simulink model "board_virgin_lab4"  (R2015a)
settings: Solver=ode3  StartTime=0.0  StopTime=inf  FixedStep=0.001  RelTol=1e-3
values from neighbouring files (symbols this model uses):
  PID_sim = PID(12)    [callback.m]    (also in postproc_lab04.m = PID(PID_idx(ii)))
  ref_2 = [0 0]    [callback.m]
  ref_3 = [0.09 0.07]    [callback.m]
  T1gain = Pt1(1)    [callback.m]
  T1offset = Pt1(2)    [callback.m]
  T2gain = Pt2(1)    [callback.m]
  T2offset = Pt2(2)    [callback.m]
  Xgain = Px(1)    [callback.m]
  Xoffset = Px(2)    [callback.m]
  Xtare_raw = [870 1250 2036 2836 3410]    [callback.m]
  Xtare_real = [-127.5 -80 0 80 127.5] * 1e-3    [callback.m]
  Ygain = Py(1)    [callback.m]
  Yoffset = Py(2)    [callback.m]
  Ytare_raw = [890 1370 2040 2690 3409]    [callback.m]
  Ytare_real = [-97.5 -50 0 50 110]*1e-3    [callback.m]
libraries: PoliArd x14, simulink x6, simulink_extras x1, dspsigops x1
settings Model: ExtModeTrigDuration=2  Creator=User  LastModifiedBy=user
settings OptimizationCC: OptimizeModelRefInitCode=on  LifeSpan=1
settings DebuggingCC: UnderspecifiedInitializationDetection=Classic  MergeDetectMultiDrivingBlocksExec=none
settings HardwareCC: ProdLargestAtomicInteger=Long  ProdLargestAtomicFloat=Double  ProdEndianess=LittleEndian  ProdHWDeviceType=ARM Compatible->ARM Cortex
settings RTWCC: SystemTargetFile=realtime.tlc  GenerateMakefile=off  TemplateMakefile=realtime.tmf  Description=Run on Target Hardware  RTWVerbose=off
settings ERTTargetCC: CombineOutputUpdateFcns=off  ExtModeTransport=3  ExtModeMexFile=ext_serial_win32_comm_rtt  ExtModeMexArgs=0 1 9600  InlinedParameterPlacement=Hierarchical  ERTSrcFileBannerTemplate=realtime_code_template.cgt  ERTHdrFileBannerTemplate=realtime_code_template.cgt  ERTDataSrcFileTemplate=realtime_code_template.cgt  ERTDataHdrFileTemplate=realtime_code_template.cgt  ERTCustomFileTemplate=realtime_file_process.tlc

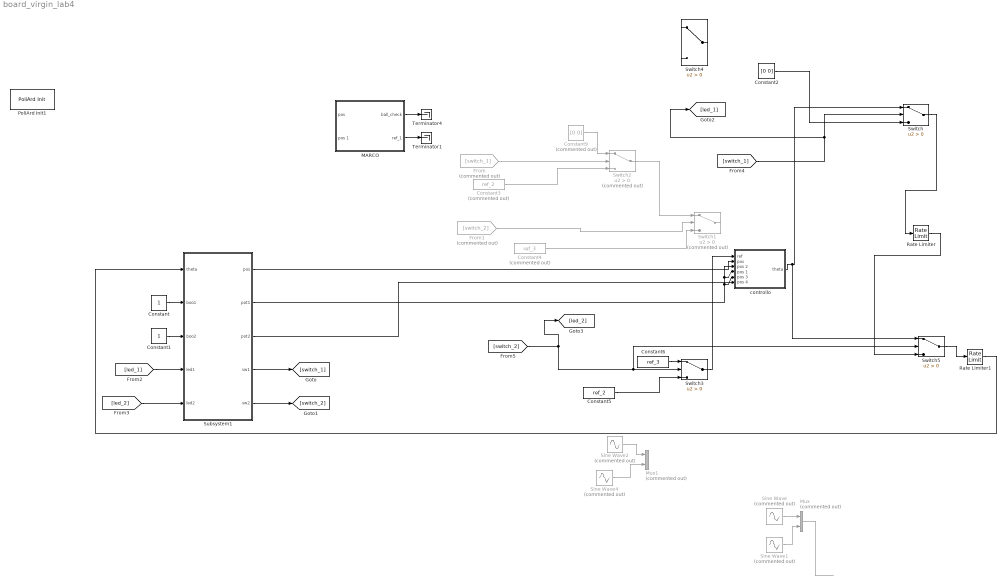
== system board_virgin_lab4 ==
  Constant : Constant  SampleTime=0.01
  Constant1 : Constant  SampleTime=0.01
  Constant2 : Constant  Value=[0 0]
  Constant3 : Constant  Commented=on  Value=ref_2
  Constant4 : Constant  Commented=on  Value=ref_3
  Constant5 : Constant  Value=ref_2
  Constant6 : Constant  Value=ref_3
  Constant9 : Constant  Commented=on  Value=[0 0]
  From : From  Commented=on  GotoTag=switch_1
  From1 : From  Commented=on  GotoTag=switch_2
  MARCO : Subsystem
  Mux : Mux  Commented=on  Inputs=2
  Mux1 : Mux  Commented=on  Inputs=2
  PoliArd Init1 : PoliArd/PoliArd Init
  Rate Limiter : RateLimiter  RisingSlewLimit=20  FallingSlewLimit=-20  SampleTimeMode=inherited
  Rate Limiter1 : RateLimiter  RisingSlewLimit=20  FallingSlewLimit=-20  SampleTimeMode=inherited
  Sine Wave : Sin  Commented=on  SampleTime=0
  Sine Wave1 : Sin  Commented=on  Phase=pi/2  SampleTime=0
  Sine Wave2 : Sin  Commented=on  Amplitude=0.03  Frequency=2*pi*0.1  SampleTime=0
  Sine Wave4 : Sin  Commented=on  Amplitude=0.03  Frequency=2*pi*0.1  Phase=pi/2  SampleTime=0
  Subsystem1 : Subsystem
  Switch{,3..5} (4 alike) : Switch  Criteria=u2 > Threshold
  Switch1 : Switch  Commented=on  Criteria=u2 > Threshold
  Switch2 : Switch  Commented=on  Criteria=u2 > Threshold
  Terminator1 : Terminator
  Terminator4 : Terminator
  "controllo " : Subsystem  SystemSampleTime=0.01
  wires:
  Subsystem1/1("pos ") -> "controllo "/2("pos ")
  Subsystem1/4(sw1) -> [switch_1]
  Subsystem1/5(sw2) -> [switch_2]
  From/1 -> Switch2/2
  From1/1 -> Switch1/2
  Constant4/1 -> Switch1/3
  [led_1] -> Subsystem1/4("led1 ")
  Constant/1 -> Subsystem1/2(boo1)
  Constant1/1 -> Subsystem1/3(boo2)
  [led_2] -> Subsystem1/5(led2)
  Constant3/1 -> Switch2/3
  Switch2/1 -> Switch1/1
  MARCO/2(ref_1) -> Terminator1/1
  Constant9/1 -> Switch2/1
  [switch_1] -> Switch/2, [led_1]
  MARCO/1(ball_check) -> Terminator4/1
  Constant2/1 -> Switch/3
  "controllo "/1(theta) -> Switch5/1, Switch/1
  Switch/1 -> Rate Limiter/1
  [switch_2] -> [led_2], Switch5/2, Switch3/2
  Constant5/1 -> Switch3/3
  Switch3/1 -> "controllo "/1("ref ")
  Rate Limiter/1 -> Switch5/3
  Switch5/1 -> Rate Limiter1/1
  Rate Limiter1/1 -> Subsystem1/1(theta)
  Mux/1 -> ?
  Sine Wave/1 -> Mux/1
  Sine Wave1/1 -> Mux/2
  Subsystem1/2(pot1) -> "controllo "/4(pos 1), "controllo "/3(pos 2), "controllo "/5(pos 3)
  Subsystem1/3(pot2) -> "controllo "/6(pos 4)
  Sine Wave2/1 -> Mux1/1
  Sine Wave4/1 -> Mux1/2
  Constant6/1 -> Switch3/1

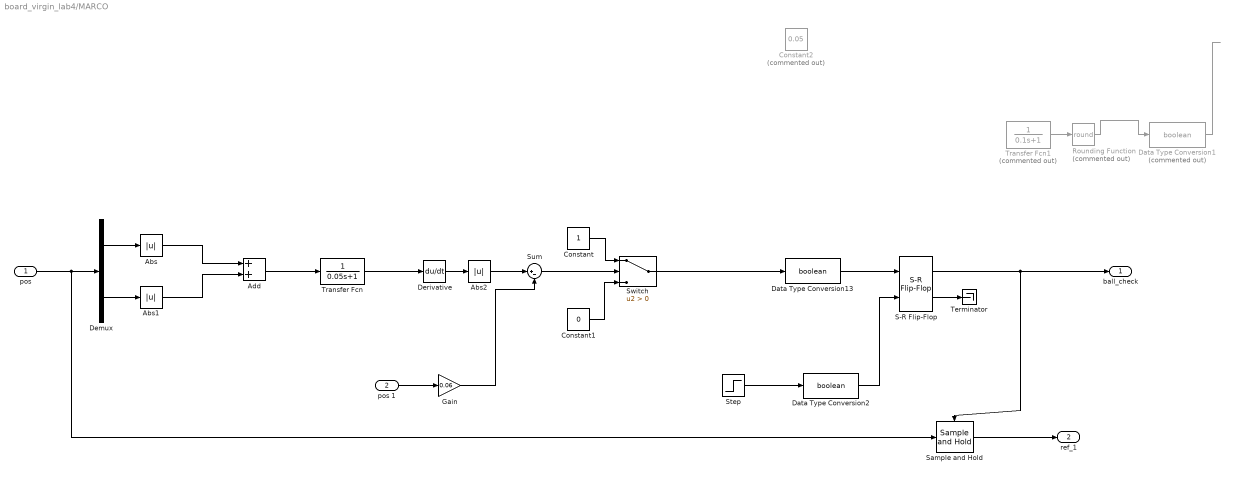
== system board_virgin_lab4/MARCO ==
  "pos " : Inport
  pos 1 : Inport  Port=2
  Abs : Abs
  Abs1 : Abs
  Abs2 : Abs
  Add : Sum
  Constant : Constant
  Constant1 : Constant  Value=0
  Constant2 : Constant  Commented=on  Value=0.05
  Data Type Conversion1 : DataTypeConversion  Commented=on  OutDataTypeStr=boolean
  Data Type Conversion13 : DataTypeConversion  OutDataTypeStr=boolean
  Data Type Conversion2 : DataTypeConversion  OutDataTypeStr=boolean
  Demux : Demux  Outputs=2
  Derivative : Derivative
  Gain : Gain  Gain=0.06
  Rounding Function : Rounding  Commented=on  Operator=round
  S-R Flip-Flop : simulink_extras/Flip Flops/S-R Flip-Flop  initial_condition=0
  Sample and Hold : dspsigops/Sample and Hold  trig=Rising edge  initCond=0  latchinput=off
  Step : Step  Before=1  After=0
  Sum : Sum  Inputs=|+-
  Switch : Switch  Criteria=u2 > Threshold
  Terminator : Terminator
  Transfer Fcn : TransferFcn  Denominator=[0.05 1]
  Transfer Fcn1 : TransferFcn  Commented=on  Denominator=[0.1 1]
  ball_check : Outport
  ref_1 : Outport  Port=2
  wires:
  "pos "/1 -> Sample and Hold/1, Demux/1
  Demux/1 -> Abs/1
  Demux/2 -> Abs1/1
  Abs1/1 -> Add/2
  Abs/1 -> Add/1
  Derivative/1 -> Abs2/1
  Abs2/1 -> Sum/1
  Sum/1 -> Switch/2
  Constant/1 -> Switch/1
  Constant1/1 -> Switch/3
  Sample and Hold/1 -> ref_1/1
  Add/1 -> Transfer Fcn/1
  Transfer Fcn/1 -> Derivative/1
  Gain/1 -> Sum/2
  S-R Flip-Flop/1 -> ball_check/1, Sample and Hold/Trigger
  S-R Flip-Flop/2 -> Terminator/1
  Data Type Conversion13/1 -> S-R Flip-Flop/1
  Switch/1 -> Data Type Conversion13/1
  Transfer Fcn1/1 -> Rounding Function/1
  Rounding Function/1 -> Data Type Conversion1/1
  ? -> Transfer Fcn1/1
  Data Type Conversion1/1 -> ?
  Data Type Conversion2/1 -> S-R Flip-Flop/2
  Step/1 -> Data Type Conversion2/1
  pos 1/1 -> Gain/1

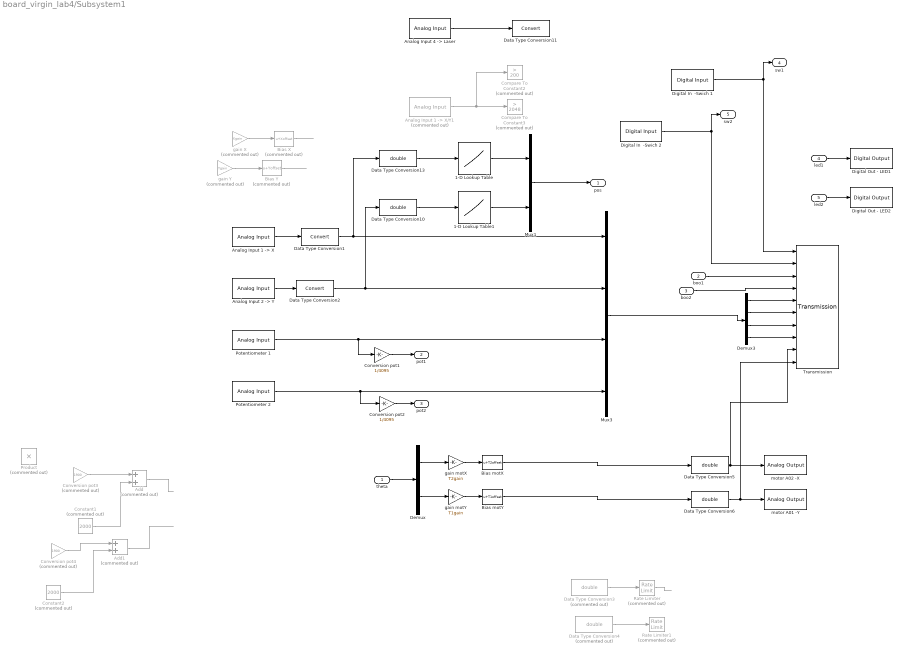
== system board_virgin_lab4/Subsystem1 ==
  theta : Inport
  boo1 : Inport  Port=2
  boo2 : Inport  Port=3
  "led1 " : Inport  Port=4
  led2 : Inport  Port=5
  1-D Lookup Table : Lookup_n-D  NumberOfTableDimensions=1  BreakpointsForDimension1=Xtare_raw  Table=Xtare_real  InternalRulePriority=Speed  RndMeth=Simplest  InputSameDT=on
  1-D Lookup Table1 : Lookup_n-D  NumberOfTableDimensions=1  BreakpointsForDimension1=Ytare_raw  Table=Ytare_real  InternalRulePriority=Speed  RndMeth=Simplest  InputSameDT=on
  Add : Sum  Commented=on
  Add1 : Sum  Commented=on
  "Analog Input 1 -> X" : PoliArd/Analog Input  AIpin_mask=1  AIsample=-1
  "Analog Input 1 -> X/Y1" : PoliArd/Analog Input  Commented=on  AIpin_mask=7  AIsample=-1
  "Analog Input 2 -> Y" : PoliArd/Analog Input  AIpin_mask=2  AIsample=-1
  "Analog Input 4 -> Laser" : PoliArd/Analog Input  AIpin_mask=4  AIsample=-1
  Bias X : Bias  Commented=on  Bias=Xoffset
  Bias Y : Bias  Commented=on  Bias=Yoffset
  Bias motX : Bias  Bias=T2offset
  Bias motY : Bias  Bias=T1offset
  Compare To Constant2 : simulink/Logic and Bit Operations/Compare To Constant  Commented=on  relop=>  const=200  OutDataTypeStr=boolean
  Compare To Constant3 : simulink/Logic and Bit Operations/Compare To Constant  Commented=on  relop=>  const=2048  OutDataTypeStr=boolean
  Constant1 : Constant  Commented=on  Value=2000
  Constant2 : Constant  Commented=on  Value=2000
  Conversion pot1 : Gain  Gain=1/4095
  Conversion pot2 : Gain  Gain=1/4095
  Conversion pot3 : Gain  Commented=on  Gain=1900
  Conversion pot4 : Gain  Commented=on  Gain=1900
  Data Type Conversion1 : DataTypeConversion
  Data Type Conversion{5..6,10,13} (4 alike) : DataTypeConversion  OutDataTypeStr=double
  Data Type Conversion11 : DataTypeConversion
  Data Type Conversion2 : DataTypeConversion
  Data Type Conversion3 : DataTypeConversion  Commented=on  OutDataTypeStr=double
  Data Type Conversion4 : DataTypeConversion  Commented=on  OutDataTypeStr=double
  Demux : Demux  Outputs=2
  Demux3 : Demux
  Digital In  -Swich 1 : PoliArd/Digital Input  DI_pin=2  DIsample=-1
  Digital In  -Swich 2 : PoliArd/Digital Input  DI_pin=3  DIsample=-1
  Digital Out - LED1 : PoliArd/Digital Output  DO_pin=1
  Digital Out - LED2 : PoliArd/Digital Output  DO_pin=2
  Mux1 : Mux  Inputs=2
  Mux3 : Mux
  Potentiometer 1 : PoliArd/Analog Input  AIpin_mask=8  AIsample=-1
  Potentiometer 2 : PoliArd/Analog Input  AIpin_mask=9  AIsample=-1
  Product : Product  Commented=on
  Rate Limiter : RateLimiter  Commented=on  RisingSlewLimit=10  FallingSlewLimit=-10  SampleTimeMode=inherited
  Rate Limiter1 : RateLimiter  Commented=on  RisingSlewLimit=10  FallingSlewLimit=-10  SampleTimeMode=inherited
  Transmission : PoliArd/Transmission  sample_freq=100  sig_to_send=6
  gain X : Gain  Commented=on  Gain=Xgain
  gain Y : Gain  Commented=on  Gain=Ygain
  gain motX : Gain  Gain=T2gain
  gain motY : Gain  Gain=T1gain
  motor A01 -Y : PoliArd/Analog Output  DAC_pin_mask=2
  motor A02 -X : PoliArd/Analog Output  DAC_pin_mask=1
  "pos " : Outport
  pot1 : Outport  Port=2
  pot2 : Outport  Port=3
  sw1 : Outport  Port=4
  sw2 : Outport  Port=5
  wires:
  "Analog Input 4 -> Laser"/1 -> Data Type Conversion11/1
  Demux3/3 -> Transmission/7
  Demux3/1 -> Transmission/5
  Demux3/2 -> Transmission/6
  "Analog Input 1 -> X/Y1"/1 -> Compare To Constant3/1, Compare To Constant2/1
  Conversion pot2/1 -> pot2/1
  Potentiometer 2/1 -> Mux3/4, Conversion pot2/1
  Conversion pot1/1 -> pot1/1
  Potentiometer 1/1 -> Conversion pot1/1, Mux3/3
  boo1/1 -> Transmission/3
  boo2/1 -> Transmission/4
  "led1 "/1 -> Digital Out - LED1/1
  led2/1 -> Digital Out - LED2/1
  Mux1/1 -> "pos "/1
  "Analog Input 1 -> X"/1 -> Data Type Conversion1/1
  "Analog Input 2 -> Y"/1 -> Data Type Conversion2/1
  Digital In  -Swich 1/1 -> Transmission/1, sw1/1
  Digital In  -Swich 2/1 -> sw2/1, Transmission/2
  Data Type Conversion1/1 -> Data Type Conversion13/1, Mux3/1
  Data Type Conversion2/1 -> Data Type Conversion10/1, Mux3/2
  gain motX/1 -> Bias motX/1
  gain motY/1 -> Bias motY/1
  Demux/1 -> gain motX/1
  Demux/2 -> gain motY/1
  theta/1 -> Demux/1
  Demux3/4 -> Transmission/8
  ? -> Conversion pot4/1
  ? -> Conversion pot3/1
  Add/1 -> ?
  Conversion pot3/1 -> Add/1
  Constant1/1 -> Add/2
  Add1/1 -> ?
  Constant2/1 -> Add1/2
  Conversion pot4/1 -> Add1/1
  Bias motY/1 -> Data Type Conversion6/1
  Data Type Conversion5/1 -> motor A02 -X/1, Transmission/9
  Data Type Conversion6/1 -> Transmission/10, motor A01 -Y/1
  Bias motX/1 -> Data Type Conversion5/1
  Data Type Conversion3/1 -> Rate Limiter/1
  Rate Limiter/1 -> ?
  Data Type Conversion4/1 -> Rate Limiter1/1
  gain X/1 -> Bias X/1
  ? -> gain X/1
  Bias X/1 -> ?
  gain Y/1 -> Bias Y/1
  ? -> gain Y/1
  Bias Y/1 -> ?
  Data Type Conversion13/1 -> 1-D Lookup Table/1
  1-D Lookup Table/1 -> Mux1/1
  Data Type Conversion10/1 -> 1-D Lookup Table1/1
  1-D Lookup Table1/1 -> Mux1/2
  Mux3/1 -> Demux3/1

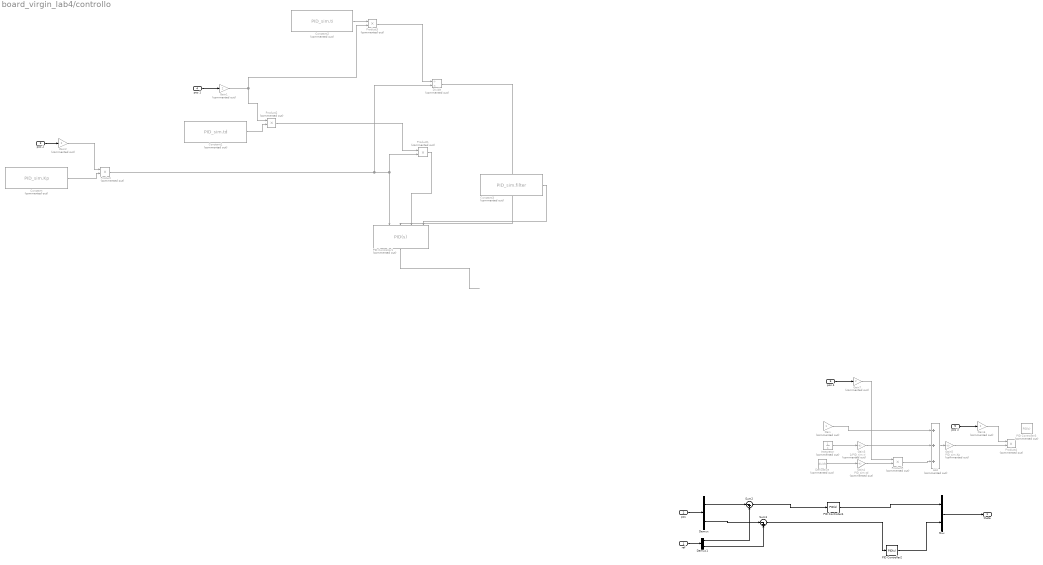
== system board_virgin_lab4/controllo  ==
  "ref " : Inport
  "pos " : Inport  Port=2
  pos 2 : Inport  Port=3
  pos 1 : Inport  Port=4
  pos 3 : Inport  Port=5
  pos 4 : Inport  Port=6
  Add : Sum  Commented=on  Inputs=+++
  Constant : Constant  Commented=on  Value=PID_sim.Kp
  Constant1 : Constant  Commented=on  Value=PID_sim.td
  Constant2 : Constant  Commented=on  Value=PID_sim.ti
  Constant3 : Constant  Commented=on  Value=PID_sim.filter
  Demux : Demux  Outputs=2
  Demux1 : Demux  Outputs=2
  Derivative : Derivative  Commented=on  CoefficientInTFapproximation=500
  Divide : Product  Commented=on  Inputs=/*
  Gain : Gain  Commented=on
  Gain{1..2,6..7} (4 alike) : Gain  Commented=on  Gain=2
  Gain3 : Gain  Commented=on  Gain=1/PID_sim.ti
  Gain4 : Gain  Commented=on  Gain=PID_sim.td
  Gain5 : Gain  Commented=on  Gain=PID_sim.Kp
  Integrator : Integrator  Commented=on
  Mux : Mux  Inputs=2
  PID Controller1 : simulink/Continuous/PID Controller  Commented=on  Controller=PID  TimeDomain=Continuous-time  SampleTime=-1  IntegratorMethod=Forward Euler  FilterMethod=Forward Euler  Form=Parallel  UseFilter=on  ControllerParametersSource=external  P=PID_sim.Kp  I=PID_sim.Ki  D=PID_sim.Kd  N=PID_sim.filter  InitialConditionSource=internal  InitialConditionForIntegrator=0  InitialConditionForFilter=0  ExternalReset=none  LimitOutput=off  UpperSaturationLimit=inf  LowerSaturationLimit=-inf  LinearizeAsGain=on  AntiWindupMode=none  Kb=1  TrackingMode=off  Kt=1  PParamMin=[]  PParamMax=[]  IParamMin=[]  IParamMax=[]  DParamMin=[]  DParamMax=[]  NParamMin=[]  NParamMax=[]  KbParamMin=[]  KbParamMax=[]  KtParamMin=[]  KtParamMax=[]  POutMin=[]  POutMax=[]  IOutMin=[]  IOutMax=[]  DOutMin=[]  DOutMax=[]  NOutMin=[]  NOutMax=[]  KbOutMin=[]  KbOutMax=[]  KtOutMin=[]  KtOutMax=[]  IntegratorOutMin=[]  IntegratorOutMax=[]  FilterOutMin=[]  FilterOutMax=[]  SumOutMin=[]  SumOutMax=[]  SumI1OutMin=[]  SumI1OutMax=[]  SumI2OutMin=[]  SumI2OutMax=[]  SumI3OutMin=[]  SumI3OutMax=[]  SumDOutMin=[]  SumDOutMax=[]  SaturationOutMin=[]  SaturationOutMax=[]  IntegratorContinuousStateAttributes=''  IntegratorStateMustResolveToSignalObject=off  IntegratorRTWStateStorageClass=Auto  FilterContinuousStateAttributes=''  FilterStateMustResolveToSignalObject=off  FilterRTWStateStorageClass=Auto  DifferentiatorICPrevScaledInput=0  DifferentiatorOutMin=[]  DifferentiatorOutMax=[]
  PID Controller2 : simulink/Continuous/PID Controller  Controller=PID  TimeDomain=Continuous-time  SampleTime=-1  IntegratorMethod=Forward Euler  FilterMethod=Forward Euler  Form=Parallel  UseFilter=off  ControllerParametersSource=internal  P=PID_sim.Kp  I=PID_sim.Ki  D=PID_sim.Kd  N=PID_sim.filter  InitialConditionSource=internal  InitialConditionForIntegrator=0  InitialConditionForFilter=0  ExternalReset=none  LimitOutput=off  UpperSaturationLimit=inf  LowerSaturationLimit=-inf  LinearizeAsGain=on  AntiWindupMode=none  Kb=1  TrackingMode=off  Kt=1  PParamMin=[]  PParamMax=[]  IParamMin=[]  IParamMax=[]  DParamMin=[]  DParamMax=[]  NParamMin=[]  NParamMax=[]  KbParamMin=[]  KbParamMax=[]  KtParamMin=[]  KtParamMax=[]  POutMin=[]  POutMax=[]  IOutMin=[]  IOutMax=[]  DOutMin=[]  DOutMax=[]  NOutMin=[]  NOutMax=[]  KbOutMin=[]  KbOutMax=[]  KtOutMin=[]  KtOutMax=[]  IntegratorOutMin=[]  IntegratorOutMax=[]  FilterOutMin=[]  FilterOutMax=[]  SumOutMin=[]  SumOutMax=[]  SumI1OutMin=[]  SumI1OutMax=[]  SumI2OutMin=[]  SumI2OutMax=[]  SumI3OutMin=[]  SumI3OutMax=[]  SumDOutMin=[]  SumDOutMax=[]  SaturationOutMin=[]  SaturationOutMax=[]  IntegratorContinuousStateAttributes=''  IntegratorStateMustResolveToSignalObject=off  IntegratorRTWStateStorageClass=Auto  FilterContinuousStateAttributes=''  FilterStateMustResolveToSignalObject=off  FilterRTWStateStorageClass=Auto  DifferentiatorICPrevScaledInput=0  DifferentiatorOutMin=[]  DifferentiatorOutMax=[]
  PID Controller3 : simulink/Continuous/PID Controller  Commented=on  Controller=PID  TimeDomain=Continuous-time  SampleTime=-1  IntegratorMethod=Forward Euler  FilterMethod=Forward Euler  Form=Parallel  UseFilter=on  ControllerParametersSource=internal  P=20  I=10  D=30  N=10  InitialConditionSource=internal  InitialConditionForIntegrator=0  InitialConditionForFilter=0  ExternalReset=none  LimitOutput=off  UpperSaturationLimit=inf  LowerSaturationLimit=-inf  LinearizeAsGain=on  AntiWindupMode=none  Kb=1  TrackingMode=off  Kt=1  PParamMin=[]  PParamMax=[]  IParamMin=[]  IParamMax=[]  DParamMin=[]  DParamMax=[]  NParamMin=[]  NParamMax=[]  KbParamMin=[]  KbParamMax=[]  KtParamMin=[]  KtParamMax=[]  POutMin=[]  POutMax=[]  IOutMin=[]  IOutMax=[]  DOutMin=[]  DOutMax=[]  NOutMin=[]  NOutMax=[]  KbOutMin=[]  KbOutMax=[]  KtOutMin=[]  KtOutMax=[]  IntegratorOutMin=[]  IntegratorOutMax=[]  FilterOutMin=[]  FilterOutMax=[]  SumOutMin=[]  SumOutMax=[]  SumI1OutMin=[]  SumI1OutMax=[]  SumI2OutMin=[]  SumI2OutMax=[]  SumI3OutMin=[]  SumI3OutMax=[]  SumDOutMin=[]  SumDOutMax=[]  SaturationOutMin=[]  SaturationOutMax=[]  IntegratorContinuousStateAttributes=''  IntegratorStateMustResolveToSignalObject=off  IntegratorRTWStateStorageClass=Auto  FilterContinuousStateAttributes=''  FilterStateMustResolveToSignalObject=off  FilterRTWStateStorageClass=Auto  DifferentiatorICPrevScaledInput=0  DifferentiatorOutMin=[]  DifferentiatorOutMax=[]
  PID Controller4 : simulink/Continuous/PID Controller  Controller=PID  TimeDomain=Continuous-time  SampleTime=-1  IntegratorMethod=Forward Euler  FilterMethod=Forward Euler  Form=Parallel  UseFilter=off  ControllerParametersSource=internal  P=PID_sim.Kp  I=PID_sim.Ki  D=PID_sim.Kd  N=PID_sim.filter  InitialConditionSource=internal  InitialConditionForIntegrator=0  InitialConditionForFilter=0  ExternalReset=none  LimitOutput=off  UpperSaturationLimit=inf  LowerSaturationLimit=-inf  LinearizeAsGain=on  AntiWindupMode=none  Kb=1  TrackingMode=off  Kt=1  PParamMin=[]  PParamMax=[]  IParamMin=[]  IParamMax=[]  DParamMin=[]  DParamMax=[]  NParamMin=[]  NParamMax=[]  KbParamMin=[]  KbParamMax=[]  KtParamMin=[]  KtParamMax=[]  POutMin=[]  POutMax=[]  IOutMin=[]  IOutMax=[]  DOutMin=[]  DOutMax=[]  NOutMin=[]  NOutMax=[]  KbOutMin=[]  KbOutMax=[]  KtOutMin=[]  KtOutMax=[]  IntegratorOutMin=[]  IntegratorOutMax=[]  FilterOutMin=[]  FilterOutMax=[]  SumOutMin=[]  SumOutMax=[]  SumI1OutMin=[]  SumI1OutMax=[]  SumI2OutMin=[]  SumI2OutMax=[]  SumI3OutMin=[]  SumI3OutMax=[]  SumDOutMin=[]  SumDOutMax=[]  SaturationOutMin=[]  SaturationOutMax=[]  IntegratorContinuousStateAttributes=''  IntegratorStateMustResolveToSignalObject=off  IntegratorRTWStateStorageClass=Auto  FilterContinuousStateAttributes=''  FilterStateMustResolveToSignalObject=off  FilterRTWStateStorageClass=Auto  DifferentiatorICPrevScaledInput=0  DifferentiatorOutMin=[]  DifferentiatorOutMax=[]
  Product{,1..5} (6 alike) : Product  Commented=on
  Sum2 : Sum  Inputs=|-+
  Sum3 : Sum  Inputs=|-+
  theta : Outport
  wires:
  "ref "/1 -> Demux1/1
  "pos "/1 -> Demux/1
  Mux/1 -> theta/1
  Demux/1 -> Sum2/1
  Demux/2 -> Sum3/1
  Demux1/1 -> Sum2/2
  Demux1/2 -> Sum3/2
  Sum3/1 -> PID Controller2/1
  PID Controller2/1 -> Mux/2
  ? -> ?
  Constant/1 -> Product/2
  pos 2/1 -> Gain2/1
  Product/1 -> Divide/2, Product1/2, PID Controller1/2
  pos 1/1 -> Gain1/1
  Constant1/1 -> Product2/2
  Gain1/1 -> Product2/1, Product3/2
  Gain2/1 -> Product/1
  Product2/1 -> Product1/1
  Constant2/1 -> Product3/1
  Product3/1 -> Divide/1
  Constant3/1 -> PID Controller1/5
  Divide/1 -> PID Controller1/3
  Product1/1 -> PID Controller1/4
  ? -> PID Controller1/1
  PID Controller1/1 -> ?
  Integrator/1 -> Gain3/1
  Derivative/1 -> Gain4/1
  Gain/1 -> Add/1
  Add/1 -> Gain5/1
  pos 3/1 -> Gain6/1
  Gain6/1 -> Product4/1
  Gain5/1 -> Product4/2
  pos 4/1 -> Gain7/1
  Gain3/1 -> Add/2
  Gain7/1 -> Product5/1
  Gain4/1 -> Product5/2
  Product5/1 -> Add/3
  Sum2/1 -> PID Controller4/1
  PID Controller4/1 -> Mux/1
